simulink model "ClosedLoopControl"  (R2016b)
settings: Solver=FixedStepDiscrete  StartTime=0.0  StopTime=Inf  FixedStep=sCoreParams.core.stepPeriod  RelTol=1e-3  EnableMultiTasking=on
undefined symbols (not defined in the file): fdesignblkfcn, gcbh, High, sCoreParams, sCoreParams_decoders_chanceDetector_randStimEventsPerSec, sCoreParams_decoders_txDetector_channel1, sCoreParams_decoders_txDetector_channel2, sCoreParams_decoders_txDetector_detectChannelInds, sCoreParams_decoders_txDetector_nChannels, sCoreParams_Features_Baseline_initialThresholdValue, sCoreParams_Features_Baseline_weightPreviousThreshold, sCoreParams_Features_Data_SmoothWindowsDurationSamples, sCoreParams_stimulator_stimAfterDelaySteps
libraries: dsparch4 x20, dspstat3 x19, dspspect3 x6, dspfdesign x2, dspindex x2, dspswit3 x1
(part 5 of 6)

== system ClosedLoopControl/FilterBanks/Variant FILTER 2000/15-30Hz Beta IIR ==
  EEGData : Inport
  Generated Filter Block : dsparch4/Biquad Filter  Tag=BlockMethodSubSystem  IIRFiltStruct=Direct form II  CoeffSource=Specify via dialog  BiQuadCoeffs=[0.03350803255605897 0 -0.03350803255605897 1 -1.968126961664987 0.97685743912432577;0.028947933140448093 0 -0.028947933140448093 1 -1.9698149829359188 0.97245132792580657;0.024518478080076195 0 -0.024518478080076195 1 -1.9433415335141357 0.94857688035351673;0.026654070338791427 0 -0.026654070338791427 1 -1.9537158945012076 0.95730690926680384;0.009247437324336031 0 -0.009247437324336031 1 -1.947476308342162 0.95468335488666101;0.024132121937224464 0 -0.024132121937224464 1 -1.9939510569744763 0.99609936563655721;0.034838789639618929 0 -0.034838789639618929 1 -1.9828610770415773 0.99197929502611926;0.018185041667705411 0 -0.018185041667705411 1 -1.961553585484159 0.96458489111915235;0.032929339024259575 0 -0.032929339024259575 1 -1.9559891723545253 0.96406022954367421;0.027829430301420995 0 -0.027829430301420995 1 -1.947222759839073 0.95155570153383873;0.034154606620126794 0 -0.034154606620126794 1 -1.9432296047878741 0.94945682008194465;0.017963086211571722 0 -0.017963086211571722 1 -1.9860735430359491 0.98829165589754697;2 0 -2 1 -1.9780358524597892 0.98041047425756744]  a0Flag=Warning  IC=0  ICnum=0  ICden=0  InputProcessing=Columns as channels (frame based)  denAccumFracLength=30  denProdOutputFracLength=30  secondMemoryFracLength=15  roundingMode=Floor  overflowMode=off  ScaleValues=[0.0021559089024979503;1;1;1;1;1;1;1;1;1;1;1;1;5.0906571453671496]  optimizeScaleValues=off  ScaleValueMode=Specify via input port (g)  scaleValueFracLength=14  FilterSource=Specify via dialog  FilterObject=BQF
  filteredData : Outport
  wires:
  EEGData/1 -> Generated Filter Block/1
  Generated Filter Block/1 -> filteredData/1

== system ClosedLoopControl/FilterBanks/Variant FILTER 2000/30-110Hz Gamma ==
  EEGData : Inport
  Generated Filter Block : dsparch4/Biquad Filter  Tag=BlockMethodSubSystem  IIRFiltStruct=Direct form II  CoeffSource=Specify via dialog  BiQuadCoeffs=[0.44494108507385505 0 -0.44494108507385505 1 -1.9229492347483501 0.93507135713401424;0.10532143902267214 0 -0.10532143902267214 1 -1.8105425689216448 0.9172820807392903;0.17172440624916194 0 -0.17172440624916194 1 -1.7910900539124941 0.81607312516795272;0.13457239531896306 0 -0.13457239531896306 1 -1.7136496566597006 0.79593164491621327;0.1225586127596065 0 -0.1225586127596065 1 -1.7279716056432983 0.768722033250546;0.10976600926481875 0 -0.10976600926481875 1 -1.6982843659738398 0.75990014481603352;0.084815037791546949 0 -0.084815037791546949 1 -1.8528164588477307 0.86967985800129866;0.11076889246798352 0 -0.11076889246798352 1 -1.7694119489785414 0.86924534061355663;0.013704961309986965 0 -0.013704961309986965 1 -1.9798873260144307 0.99084807550474052;0.043836861216569364 0 -0.043836861216569364 1 -1.9615194301123848 0.97260947934511921;0.056396566360770645 0 -0.056396566360770645 1 -1.9018156854278072 0.91495586562429665;0.14612631243940441 0 -0.14612631243940441 1 -1.8786742611057465 0.89332221918518917;0.31121173058758267 0 -0.31121173058758267 1 -1.7575331753835428 0.78939937275597161;0.22500607059927488 0 -0.22500607059927488 1 -1.700551481385171 0.77274372032905814;0.089481111718450551 0 -0.089481111718450551 1 -1.7074644298185397 0.75840447453517756;0.38286644242384676 0 -0.38286644242384676 1 -1.8235966810827047 0.84373660447540921;0.21166451671099704 0 -0.21166451671099704 1 -1.7368477683794912 0.8284349024879869;0.049747984077454795 0 -0.049747984077454795 1 -1.8592586643974909 0.97126523399925213;2 0 -2 1 -1.9426828814559494 0.95414675458837162]  a0Flag=Warning  IC=0  ICnum=0  ICden=0  InputProcessing=Columns as channels (frame based)  denAccumFracLength=30  denProdOutputFracLength=30  secondMemoryFracLength=15  roundingMode=Floor  overflowMode=off  ScaleValues=[0.0069254201507007191;1;1;1;1;1;1;1;1;1;1;1;1;1;1;1;1;1;1;2.245698055179957]  optimizeScaleValues=off  ScaleValueMode=Specify via input port (g)  scaleValueFracLength=14  FilterSource=Specify via dialog  FilterObject=BQF
  filteredData : Outport
  wires:
  EEGData/1 -> Generated Filter Block/1
  Generated Filter Block/1 -> filteredData/1

== system ClosedLoopControl/FilterBanks/Variant FILTER 2000/30-55Hz LowGamma FIR ==
  EEGData : Inport
  Generated Filter Block : DiscreteFir  Tag=BlockMethodSubSystem  Coefficients=[0.012220426722110508 -0.012179228647942394 -0.0054004824998452744 -0.00086107993631961153 0.0018357528942907909 0.0031129006980230925 0.0033526002586839569 0.0029004097183938193 0.002025756039159722 0.00094619130244101926 -0.00019186502278131733 -0.0012796989292308341 -0.0022643735403191324 -0.0031100749332247601 -0.0038138220234182119 -0.0043728519036089321 -0.0048073661756172087 -0.0051211291794167951 -0.0053355515893745153 -0.0054503938965098165 -0.0054804722865874379 -0.0054225157087565935 -0.0052837766862496747 -0.0050558969555260557 -0.0047473427181577406 -0.0043490854638637624 -0.0038740240389517158 -0.0033141899320159045 -0.0026891371712456872 -0.0019988658326665788 -0.0012668077012148425 -0.00049777159136449409 0.00027980011654713644 0.0010569221711767803 0.0018012584862141282 0.0025073080725695955 0.0031419799261284092 0.0037039342557620781 0.0041592221536759701 0.00451661684396605 0.004753834670207643 0.004858091055885313 0.0048732693610234797 0.004719918151711854 0.004501106268126308 0.0041695525933403083 0.0037390943415244577 0.0032614183648101208 0.0027532787181978611 0.0022113037703167591 0.0016750315037899622 0.001183752691769548 0.00075535761814340149 0.00039953150366791961 0.00014046384937540252 6.1491868128734175e-06 1.1186901667634026e-05 0.00015526412697483837 0.0004330345318633678 0.00085176463289905009 0.0014052355878874233 0.0020800590767608707 0.002849623480313646 0.0036845580548849717 0.0045549014833176776 0.0054328429633881004 0.0062766851830694257 0.0070524883129054004 0.0077090516676290282 0.0082134484811023818 0.0085227769306376287 0.0086142017649426875 0.0084547786472301146 0.0080253554621038687 0.0073005963266854152 0.0062785521595116736 0.004954769987550566 0.0033487584764538918 0.0014699436712954949 -0.00064363377180517154 -0.0029663837162192072 -0.0054436946157823849 -0.0080298692849513926 -0.010667639233237229 -0.013277806853810465 -0.015812438746192266 -0.018188194707908951 -0.020345799993991307 -0.022224250296602483 -0.023753925738189897 -0.02488365206526176 -0.025570322564561061 -0.025766825493726914 -0.025444977817514449 -0.024595476521060467 -0.023213441870529743 -0.021305593868567389 -0.018898508751834929 -0.016029060137637101 -0.012740944050543842 -0.0090932386572889021 -0.0051505995714406739 -0.0009962643893293105 0.0032817393593285271 0.0076023297562782021 0.01187015497436876 0.01599167911755478 0.01987965668781326 0.023442825796413751 0.026611571958282988 0.029305287988366832 0.031470080206127349 0.033049785633532322 0.034015176943345569 0.034337823655261598 0.034015176943345569 0.033049785633532322 0.031470080206127349 0.029305287988366832 0.026611571958282988 0.023442825796413751 0.01987965668781326 0.01599167911755478 0.01187015497436876 0.0076023297562782021 0.0032817393593285271 -0.0009962643893293105 -0.0051505995714406739 -0.0090932386572889021 -0.012740944050543842 -0.016029060137637101 -0.018898508751834929 -0.021305593868567389 -0.023213441870529743 -0.024595476521060467 -0.025444977817514449 -0.025766825493726914 -0.025570322564561061 -0.02488365206526176 -0.023753925738189897 -0.022224250296602483 -0.020345799993991307 -0.018188194707908951 -0.015812438746192266 -0.013277806853810465 -0.010667639233237229 -0.0080298692849513926 -0.0054436946157823849 -0.0029663837162192072 -0.00064363377180517154 0.0014699436712954949 0.0033487584764538918 0.004954769987550566 0.0062785521595116736 0.0073005963266854152 0.0080253554621038687 0.0084547786472301146 0.0086142017649426875 0.0085227769306376287 0.0082134484811023818 0.0077090516676290282 0.0070524883129054004 0.0062766851830694257 0.0054328429633881004 0.0045549014833176776 0.0036845580548849717 0.002849623480313646 0.0020800590767608707 0.0014052355878874233 0.00085176463289905009 0.0004330345318633678 0.00015526412697483837 1.1186901667634026e-05 6.1491868128734175e-06 0.00014046384937540252 0.00039953150366791961 0.00075535761814340149 0.001183752691769548 0.0016750315037899622 0.0022113037703167591 ...(+1099 chars)]  InputProcessing=Columns as channels (frame based)
  filteredData : Outport
  wires:
  EEGData/1 -> Generated Filter Block/1
  Generated Filter Block/1 -> filteredData/1

== system ClosedLoopControl/FilterBanks/Variant FILTER 2000/30-55Hz LowGamma IIR ==
  EEGData : Inport
  Generated Filter Block : dsparch4/Biquad Filter  Tag=BlockMethodSubSystem  IIRFiltStruct=Direct form II  CoeffSource=Specify via dialog  BiQuadCoeffs=[0.054971163915039548 0 -0.054971163915039548 1 -1.9365232082566068 0.96457485704660062;0.045303454328115444 0 -0.045303454328115444 1 -1.943815405190324 0.95402280190252708;0.040876564560681977 0 -0.040876564560681977 1 -1.9021901915191075 0.92014242905657051;0.039452297008396219 0 -0.039452297008396219 1 -1.9181591402612868 0.93133725483473273;0.016797067377568437 0 -0.016797067377568437 1 -1.9071214770857949 0.93068451608425717;0.033290819682779867 0 -0.033290819682779867 1 -1.9846770422373305 0.99329244607990996;0.027940855529409586 0 -0.027940855529409586 1 -1.9583863274249822 0.98768107623138823;0.056178592840272178 0 -0.056178592840272178 1 -1.9190061246773207 0.94507958913772061;0.051950069443619865 0 -0.051950069443619865 1 -1.9304457502044112 0.94190985278343375;0.042977804135131976 0 -0.042977804135131976 1 -1.9082136337884117 0.92357824758871798;0.056640067873580391 0 -0.056640067873580391 1 -1.9015398053776527 0.92230686978965282;0.032630838991779737 0 -0.032630838991779737 1 -1.9711576392292749 0.97999233217843884;2 0 -2 1 -1.957503630091644 0.96685458848731587]  a0Flag=Warning  IC=0  ICnum=0  ICden=0  InputProcessing=Columns as channels (frame based)  denAccumFracLength=30  denProdOutputFracLength=30  secondMemoryFracLength=15  roundingMode=Floor  overflowMode=off  ScaleValues=[0.0059317819644075995;1;1;1;1;1;1;1;1;1;1;1;1;2.5603283637290581]  optimizeScaleValues=off  ScaleValueMode=Specify via input port (g)  scaleValueFracLength=14  FilterSource=Specify via dialog  FilterObject=BQF
  filteredData : Outport
  wires:
  EEGData/1 -> Generated Filter Block/1
  Generated Filter Block/1 -> filteredData/1

== system ClosedLoopControl/FilterBanks/Variant FILTER 2000/4-8Hz Theta FIR ==
  EEGData : Inport
  Generated Filter Block : DiscreteFir  Tag=BlockMethodSubSystem  Coefficients=[-4.0965914206968854e-05 -3.1562576663732106e-05 -2.1885911724999518e-05 -1.1939596349254351e-05 -1.7275529186717732e-06 8.7460521918561927e-06 1.947681025149899e-05 3.0460072015961004e-05 4.1690949775364282e-05 5.316431960704088e-05 6.4874823832640496e-05 7.6816873678724166e-05 8.8984652139878232e-05 0.00010137211704322235 0.00011397300431296607 0.00012678083143356132 0.00013978890110980167 0.00015299030512201677 0.0001663779283744122 0.00017994445313437968 0.00019368236346045136 0.00020758394981644162 0.00022164131386907284 0.00023584637346632409 0.00025019086779349122 0.00026466636270383186 0.00027926425622051192 0.00029397578420637229 0.0003087920261979428 0.00032370391139992542 0.00033870222483622773 0.00035377761365352274 0.00036892059357309124 0.00038412155548662883 0.00039937077219152613 0.00041465840526098188 0.00042997451204421873 0.00044530905279189289 0.00046065189790167919 0.00047599283527891651 0.00049132157780700891 0.00050662777092225068 0.00052190100028754523 0.00053713079955942423 0.0005523066582426813 0.00056741802962677009 0.00058245433879808891 0.000597404990722145 0.00061225937838948802 0.00062700689101926807 0.00064163692231413751 0.0006561388787601712 0.00067050218796541777 0.00068471630703058827 0.00069877073094537284 0.00071265500100379619 0.00072635871323196185 0.00073987152682152089 0.00075318317256212598 0.00076628346126611058 0.00077916229217862127 0.00079180966136635381 0.00080421567007808498 0.00081637053307013834 0.00082826458688991199 0.00083988829811062636 0.0008512322715104072 0.00086228725818885592 0.00087304416361427394 0.00088349405559469028 0.00089362817216592349 0.00090343792938986952 0.00091291492905630825 0.00092205096628152127 0.00093083803699705442 0.0009392683453220477 0.00094733431081258041 0.00095502857558154447 0.00096234401128264535 0.00096927372595218225 0.00097581107070235091 0.0009819496462598993 0.00098768330934403915 0.00099300617887762544 0.00099791264202572761 0.0010023973600557757 0.0010064552740136482 0.0010100816102101011 0.0010132718855121318 0.001016021912433947 0.0010183278040223579 0.0010201859785315629 0.001021593163882393 0.0010225464019012794 0.0010230430523343159 0.0010230807966319598 0.0010226576415000763 0.0010217719222131735 0.0010204223056858744 0.0010186077932988016 0.0010163277234752684 0.0010135817740053027 0.001010369964113756 0.0010066926562693997 0.0010025505577321177 0.00099794472183549455 0.00099287654900228565 0.00098734778749046018 0.00098136053386771059 0.00097491723321251631 0.00096802067904005952 0.00096067401295151704 0.00095288072400541532 0.0009446446478100181 0.0009359699653358561 0.00092686120144778344 0.0009173232231561401 0.00090736123758679863 0.00089698078967015025 0.00088618775954923501 0.00087498835970750667 0.00086338913181691805 0.00085139694330722165 0.00083901898365764142 0.00082626276041227885 0.00081313609492081231 0.00079964711780634835 0.00078580426416241132 0.00077161626848136554 0.0007570921593167498 0.00074224125368220961 0.00072707315118998063 0.00071159772793206099 0.00069582513010743195 0.00067976576739893664 0.00066343030610358899 0.00064682966202034113 0.00062997499309955815 0.0006128776918585834 0.00059554937756810765 0.00057800188821412754 0.00056024727224058429 0.00054229778007792984 0.00052416585546304225 0.00050586412655614986 0.00048740539686060552 0.00046880263595147945 0.00045006897001921846 0.00043121767223470618 0.00041226215294230351 0.00039321594968756213 0.00037409271708650435 0.00035490621654351472 0.0003356703058250473 0.00031639892849649162 0.00029710610322969557 0.00027780591298878944 0.00025851249410209314 0.0002392400252279985 0.00022000271622286136 0.00020081479691906072 0.00018169050582149475 0.00016264407873087066 0.00014368973730227231 0.00012484167754757907 0.00010611405829039998 8.7520989582255267e-05 6.9076521088845522e-05 5.0794630455274516e-05 3.268921165922444e-05 1.4774063361054236e-05 -2.937122740077089e-06 -2.0430773534982893e-05 -3.7693446108933282e-05 -5.4711839312708335e-05 ...(+22999 chars)]  InputProcessing=Columns as channels (frame based)
  filteredData : Outport
  wires:
  EEGData/1 -> Generated Filter Block/1
  Generated Filter Block/1 -> filteredData/1

== system ClosedLoopControl/FilterBanks/Variant FILTER 2000/4-8Hz Theta IIR ==
  EEGData : Inport
  Generated Filter Block : dsparch4/Biquad Filter  Tag=BlockMethodSubSystem  IIRFiltStruct=Direct form II  CoeffSource=Specify via dialog  BiQuadCoeffs=[0.034870161803218065 0 -0.034870161803218065 1 -1.9901820445662115 0.99030010068899088;0.009182818059100822 0 -0.009182818059100822 1 -1.987831524827155 0.98862483074806906;0.011702989635403891 0 -0.011702989635403891 1 -1.9821347784883785 0.98235114496605769;0.0012579336984153335 0 -0.0012579336984153335 1 -1.9781755212957257 0.97849733044258869;0.0019210830021429274 0 -0.0019210830021429274 1 -1.9986640854686097 0.99874844354806203;0.0076620170177267881 0 -0.0076620170177267881 1 -1.9960972294760821 0.99618605713604058;0.033863322083021209 0 -0.033863322083021209 1 -1.9864562832778709 0.98660899779358613;0.028291249228048612 0 -0.028291249228048612 1 -1.9817633511668777 0.98247167969757787;0.022295304396116152 0 -0.022295304396116152 1 -1.9777517678595222 0.97834385452484562;0.028819253989087464 0 -0.028819253989087464 1 -1.9764476095472279 0.97690415306032918;0.0044545219959124804 0 -0.0044545219959124804 1 -1.9952152592319994 0.99605478634023081;2 0 -2 1 -1.9933280019994593 0.99342704312088992]  a0Flag=Warning  IC=0  ICnum=0  ICden=0  InputProcessing=Columns as channels (frame based)  denAccumFracLength=30  denProdOutputFracLength=30  secondMemoryFracLength=15  roundingMode=Floor  overflowMode=off  ScaleValues=[9.4482396346836273e-05;1;1;1;1;1;1;1;1;1;1;1;24.883500210657072]  optimizeScaleValues=off  ScaleValueMode=Specify via input port (g)  scaleValueFracLength=14  FilterSource=Specify via dialog  FilterObject=BQF
  filteredData : Outport
  wires:
  EEGData/1 -> Generated Filter Block/1
  Generated Filter Block/1 -> filteredData/1

== system ClosedLoopControl/FilterBanks/Variant FILTER 2000/65-110Hz HighGamma FIR ==
  EEGData : Inport
  Generated Filter Block : DiscreteFir  Tag=BlockMethodSubSystem  Coefficients=[0.013804330140111717 -0.0032030301327593746 -0.0026076510316669732 -0.0019065599324483403 -0.0010950973516722739 -0.00016216284695244599 0.00086566972400229725 0.0019516885555648496 0.0030106913379105565 0.0039390669121143725 0.0046071460998753817 0.0048943907316536354 0.0046884459511977224 0.0039269229728160996 0.0025931297718577782 0.00075000967683423552 -0.0014812603255484518 -0.0039070830585515659 -0.0062985241582419948 -0.0083973498946592028 -0.0099678263784681084 -0.010809035903715401 -0.010803230740337099 -0.0099149025044472407 -0.0082222253166924462 -0.0058958474615859622 -0.0031966951596653086 -0.00042921572872034144 0.0020843075499259859 0.0040591524840028152 0.005272016533938776 0.0056235264011517839 0.0051356663591639361 0.0039469466526657771 0.0023736337698522614 0.00069406556447416045 -0.00062224964462739992 -0.0012265818590162169 -0.00086373706682174275 0.00064926343879799649 0.0032891772017854025 0.0068616007904351807 0.010959888764209976 0.015047965951643011 0.018483860601451012 0.020629088707457537 0.020895258620364673 0.018864941232038121 0.014327792052099074 0.0073683568396857536 -0.0016488647216768106 -0.012058123582057797 -0.022974047895930626 -0.033340495226029006 -0.042069205650392676 -0.048123624580120594 -0.050670829782113042 -0.04915218268598933 -0.043397073906481516 -0.033631108507841165 -0.020501148353700021 -0.0049965672361083416 0.011603807282296149 0.02788293342498982 0.042383528564973294 0.053814263792701968 0.061127840120098795 0.06363510173931633 0.061127840120098795 0.053814263792701968 0.042383528564973294 0.02788293342498982 0.011603807282296149 -0.0049965672361083416 -0.020501148353700021 -0.033631108507841165 -0.043397073906481516 -0.04915218268598933 -0.050670829782113042 -0.048123624580120594 -0.042069205650392676 -0.033340495226029006 -0.022974047895930626 -0.012058123582057797 -0.0016488647216768106 0.0073683568396857536 0.014327792052099074 0.018864941232038121 0.020895258620364673 0.020629088707457537 0.018483860601451012 0.015047965951643011 0.010959888764209976 0.0068616007904351807 0.0032891772017854025 0.00064926343879799649 -0.00086373706682174275 -0.0012265818590162169 -0.00062224964462739992 0.00069406556447416045 0.0023736337698522614 0.0039469466526657771 0.0051356663591639361 0.0056235264011517839 0.005272016533938776 0.0040591524840028152 0.0020843075499259859 -0.00042921572872034144 -0.0031966951596653086 -0.0058958474615859622 -0.0082222253166924462 -0.0099149025044472407 -0.010803230740337099 -0.010809035903715401 -0.0099678263784681084 -0.0083973498946592028 -0.0062985241582419948 -0.0039070830585515659 -0.0014812603255484518 0.00075000967683423552 0.0025931297718577782 0.0039269229728160996 0.0046884459511977224 0.0048943907316536354 0.0046071460998753817 0.0039390669121143725 0.0030106913379105565 0.0019516885555648496 0.00086566972400229725 -0.00016216284695244599 -0.0010950973516722739 -0.0019065599324483403 -0.0026076510316669732 -0.0032030301327593746 0.013804330140111717]  InputProcessing=Columns as channels (frame based)
  filteredData : Outport
  wires:
  EEGData/1 -> Generated Filter Block/1
  Generated Filter Block/1 -> filteredData/1

== system ClosedLoopControl/FilterBanks/Variant FILTER 2000/65-110Hz HighGamma IIR ==
  EEGData : Inport
  Generated Filter Block : dsparch4/Biquad Filter  Tag=BlockMethodSubSystem  IIRFiltStruct=Direct form II  CoeffSource=Specify via dialog  BiQuadCoeffs=[0.03481066597565307 0 -0.03481066597565307 1 -1.9044776337910623 0.95038435851939029;0.078431168263520465 0 -0.078431168263520465 1 -1.8838667407265433 0.9317664529692361;0.1124032550031358 0 -0.1124032550031358 1 -1.8092080071802343 0.8746503799570835;0.12760029829927499 0 -0.12760029829927499 1 -1.7851154536991634 0.87280244579405086;0.05117355277674826 0 -0.05117355277674826 1 -1.7981791696471037 0.9013800345321431;0.0084596408133775832 0 -0.0084596408133775832 1 -1.8437514040399918 0.89841797883106722;0.17610164240743503 0 -0.17610164240743503 1 -1.9453914043828053 0.98981101927967896;0.16070437686852881 0 -0.16070437686852881 1 -1.8641179377976567 0.98348433956074843;0.046051454658558776 0 -0.046051454658558776 1 -1.8144389250478108 0.92438172679701502;0.095494036627962964 0 -0.095494036627962964 1 -1.8634769576441372 0.914274980256637;0.10866980756531945 0 -0.10866980756531945 1 -1.7963849891719041 0.86863193889629275;0.064753210049586174 0 -0.064753210049586174 1 -1.7880209106179794 0.86778390972292085;0.094302543944276437 0 -0.094302543944276437 1 -1.8253592148117952 0.88490987431890045;0.022974288403234164 0 -0.022974288403234164 1 -1.7883860690659723 0.88402564354732227;0.16350969038402483 0 -0.16350969038402483 1 -1.9250396972494057 0.96979928748005073;1.9999999999999998 0 -1.9999999999999998 1 -1.8367052589315991 0.95216011987026072]  a0Flag=Warning  IC=0  ICnum=0  ICden=0  InputProcessing=Columns as channels (frame based)  denAccumFracLength=30  denProdOutputFracLength=30  secondMemoryFracLength=15  roundingMode=Floor  overflowMode=off  ScaleValues=[0.010630195163103937;1;1;1;1;1;1;1;1;1;1;1;1;1;1;1;1.1474080820014845]  optimizeScaleValues=off  ScaleValueMode=Specify via input port (g)  scaleValueFracLength=14  FilterSource=Specify via dialog  FilterObject=BQF
  filteredData : Outport
  wires:
  EEGData/1 -> Generated Filter Block/1
  Generated Filter Block/1 -> filteredData/1
